simulink model "main"  (R2024a)
settings: Solver=FixedStepDiscrete  StartTime=0.0  StopTime=5  RelTol=1e-3
PreLoadFcn:
  | RTWConfigurationCB('preloadfcn', bdroot);
model workspace (MAT data in the model file):
  fault_count = 0
undefined symbols (not defined in the file or in its folder): Call, Function
libraries: canmsglib x15, c280xlib x13, c2837xDlib x9, c2802xlib x8, simulink x4, slpidlib x1
(part 1 of 2)
settings Model: SimulationMode=external  ExtModeTrigDuration=8  Creator=Brian  LastModifiedBy=benjaminlevin
settings SolverCC: AutoInsertRateTranBlk=on
settings OptimizationCC: DefaultUnderspecifiedDataType=single  EnhancedBackFolding=on  PassReuseOutputArgsAs=Individual arguments  MaxStackSize=1024  OptimizeBlockOrder=speed  DifferentSizesBufferReuse=on  OptimizationCustomize=off  DenormalBehavior=FlushToZero  EfficientTunableParamExpr=on
settings DebuggingCC: ParameterTunabilityLossMsg=error
settings HardwareCC: ProdBitPerChar=16  ProdBitPerInt=16  ProdBitPerPointer=32  ProdBitPerSizeT=32  ProdBitPerPtrDiffT=32  ProdLargestAtomicInteger=Integer  ProdLargestAtomicFloat=None  ProdWordSize=16  ProdLongLongMode=on  ProdHWDeviceType=Texas Instruments->C2000  HardwareBoardFeatureSet=SoCBlockset
settings ModelReferenceCC: EnableRefExpFcnMdlSchedulingChecks=on  ModelReferenceNumInstancesAllowed=Single
settings SFSimCC: MATLABDynamicMemAlloc=off
settings RTWCC: Description=Embedded Coder  SystemTargetFile=ert.tlc  HardwareBoard=TI Delfino F28379D LaunchPad  TemplateMakefile=ert_default_tmf  Toolchain=Texas Instruments Code Composer Studio (C2000)  CodeProfilingSaveOptions=MetricsOnly  GPUComputeCapability=3.5
settings CodeAppCC: ForceParamTrailComments=on  IgnoreCustomStorageClasses=off  OperatorAnnotations=on  SimulinkDataObjDesc=on  SFDataObjDesc=on  InsertBlockDesc=on
settings ERTTargetCC: CodeReplacementLibrary=TI C28x  ExtModeTransport=4  ExtModeStaticAlloc=on  ExtModeAutomaticAllocSize=off  ExtModeStaticAllocSize=10000  ExtModeMexFile=ext_xcp  ExtModeIntrfLevel=Level2 - Open

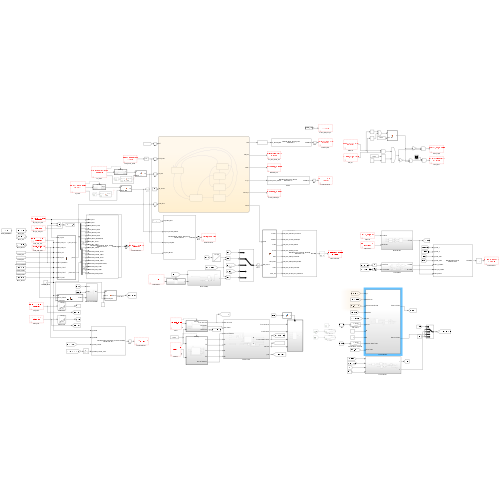
[thumbnail: Simulink's stored preview of the top-level diagram]
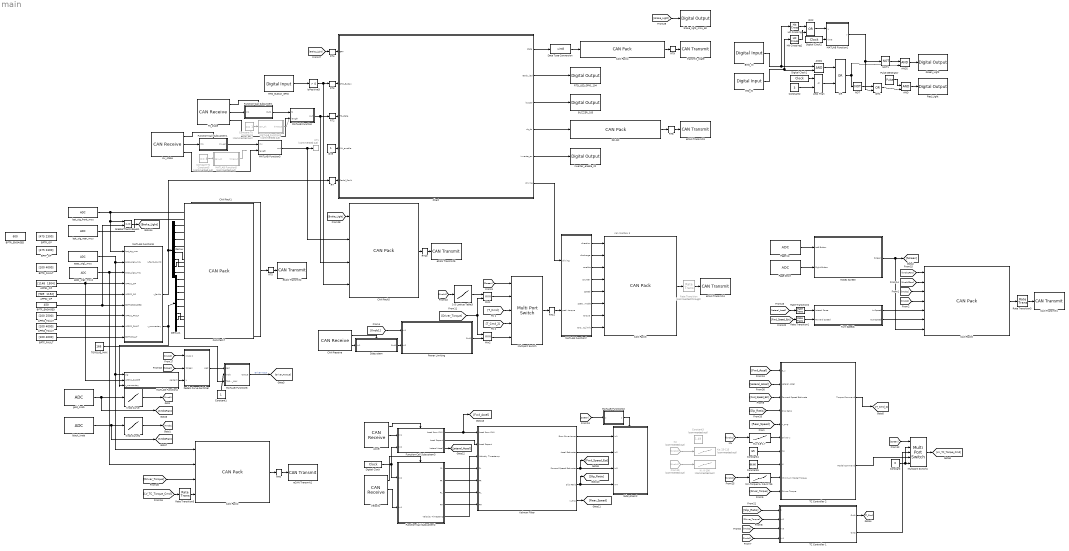
== system main ==
  note: can mailbox 3
  1-D Lookup Table3 : Lookup_n-D  NumberOfTableDimensions=1  BreakpointsForDimension1=[1;10]  Table=[0;166]  ExtrapMethod=Clip  InternalRulePriority=Speed  RndMeth=Simplest
  AND : Logic  IconShape=distinctive  AllPortsSameDT=off  OutDataTypeStr=boolean
  AND1 : Logic  IconShape=distinctive  AllPortsSameDT=off  OutDataTypeStr=boolean
  AND2 : Logic  IconShape=distinctive  AllPortsSameDT=off  OutDataTypeStr=boolean
  APPS1_FAULT : Constant  Value=[100 2500]  VectorParams1D=off
  APPS1_OP : Constant  Value="[1148  1504]"  VectorParams1D=off
  APPS2_FAULT : Constant  Value=[100 4000]  VectorParams1D=off
  APPS2_OP : Constant  Value="[989  1152]"  VectorParams1D=off
  Accel : c280xlib/CAN Receive  chipFamily=C280x  useModule=CAN_B  mailboxNo=10  messageID=52  messageType=Standard (11-bit identifier)  enableAcceptanceFiltering=off  messageIDMask=0  sampleTime=.001  dataType=CAN_MESSAGE_TYPE  outputAction=Output last received values  initValue=0  outputMessageID=off  outputMessageLength=on  outputMessageTimeStamp=off  postInterrupt=off  interruptLine=0
  BMS_IN : c2837xDlib/Digital Input  GPIO_Number=GPIO104~GPIO111  GPIO_Bit0=off  GPIO_Bit1=off  GPIO_Bit2=off  GPIO_Bit3=off  GPIO_Bit4=off  GPIO_Bit5=off  GPIO_Bit6=off  GPIO_Bit7=on  sampleTime=0.1  dataType=auto  GPIO_Bit0_Qualification=Sync to SYSCLKOUT  GPIO_Bit1_Qualification=Sync to SYSCLKOUT  GPIO_Bit2_Qualification=Sync to SYSCLKOUT  GPIO_Bit3_Qualification=Sync to SYSCLKOUT  GPIO_Bit4_Qualification=Sync to SYSCLKOUT  GPIO_Bit5_Qualification=Sync to SYSCLKOUT  GPIO_Bit6_Qualification=Sync to SYSCLKOUT  GPIO_Bit7_Qualification=Sync to SYSCLKOUT  Qualification_Period=-1
  BPTF_ENGAGED : Constant  Value=450  VectorParams1D=off
  BPTF_FAULT : Constant  Value=[100 4000]  VectorParams1D=off
  BPTF_OP : Constant  Value=[475 2300]  VectorParams1D=off
  BPTR_ENGAGED : Constant  Value=600  VectorParams1D=off
  BPTR_FAULT : Constant  Value=[100 4000]  VectorParams1D=off
  BPTR_OP : Constant  Value=[475 2300]  VectorParams1D=off
  BUZZER_105 : c2837xDlib/Digital Output  GPIO_Number=GPIO104~GPIO111  GPIO_Bit0=off  GPIO_BIT0_Toggle=off  GPIO_Bit1=on  GPIO_BIT1_Toggle=off  GPIO_Bit2=off  GPIO_BIT2_Toggle=off  GPIO_Bit3=off  GPIO_BIT3_Toggle=off  GPIO_Bit4=off  GPIO_BIT4_Toggle=off  GPIO_Bit5=off  GPIO_BIT5_Toggle=off  GPIO_Bit6=off  GPIO_BIT6_Toggle=off  GPIO_Bit7=off  GPIO_BIT7_Toggle=off
  CAN Pack1 : canmsglib/CAN Pack  MsgList=(none)  MsgName=M402_Brakes_Faults_Display  MsgIDType=Standard (11-bit identifier)  MsgIdentifier=402  MsgLength=6  Remote=off  ApplyMinMax=off  BusOutput=off  SignalInfo={'LV_BPT_Front','16','16','LE','unsigned','Standard','0','1','0','-Inf','Inf';'LV_BPT_Rear','0','16','LE','unsigned','Standard','0','1','0','-Inf','Inf';'LV_Fault_APPS1_Lower','32','1','LE','unsigned','Standard','0','1','0','0','1';'LV_Fault_APPS1_Upper','33','1','LE','unsigned','Standard','0','1','0','0','1';'LV_Fault_APPS2_Lower','34','1','LE','unsigned','Standard','0','1','0','0','1';'LV_Fault_APPS2_Upper','35','1','LE','unsigned','Standard','0','1','0','0','1';'LV_Fault_APPS_Implausibility','38','1','LE','unsigned','Standard','0','1','0','0','1';'LV_Fault_BPT_Lower','36','1','LE','unsigned','Standard','0','1','0','0','1';'LV_Fault_BPT_Upper','37','1','LE','unsigned','Standard','0','1','0','0','1';'LV_Fault_Both_Pedals','39','1','LE','unsigned','Standard','0','1','0','0','1';'LV_Momentary_APPS1_Lower','40','1','LE','unsigned','Standard','0','1','0','0','1';'LV_Momentary_APPS1_Upper','41','1','LE','unsigned','Standard','0','1','0','0','1';'LV_Momentary_APPS2_Lower','42','1','LE','unsigned','Standard','0','1','0','0','1';'LV_Momentary_APPS2_Upper','43','1','LE','unsigned','Standard','0','1','0','0','1';'LV_Momentary_APPS_Implausibility','46','1','LE','unsigned','Standard','0','1','0','0','1';'LV_Momentary_BPT_Lower','44','1','LE','unsigned','Standard','0','1','0','0','1';'LV_Momentary_BPT_Upper','45','1','LE','unsigned','Standard','0','1','0','0','1';'LV_Momentary_Both_Pedals','47','1','LE','unsigned','Standard','0','1','0','0','1'}
      settings: DataFormat=manually specified signals
  CAN Pack2 : canmsglib/CAN Pack  MsgList=(none)  MsgName=M401_Accelerator_Controls  MsgIDType=Standard (11-bit identifier)  MsgIdentifier=401  MsgLength=8  Remote=off  ApplyMinMax=off  BusOutput=off  SignalInfo={'LV_APPS1','0','16','LE','unsigned','Standard','0','1','0','0','4095';'LV_APPS2','16','16','LE','unsigned','Standard','0','1','0','0','4095';'LV_Driver_Torque','48','16','LE','signed','Standard','0','0.1','0','-3276.8','3276.7';'LV_Kalman_Torque_Cmd','32','16','LE','signed','Standard','0','0.1','0','-3276.8','3276.7'}
      settings: DataFormat=manually specified signals
  CAN Pack3 : canmsglib/CAN Pack  MsgList=(none)  MsgName=M176_Command_Message  MsgIDType=Standard (11-bit identifier)  MsgIdentifier=176  MsgLength=8  Remote=off  ApplyMinMax=off  BusOutput=off  SignalInfo={'VCU_INV_Direction_Command','32','1','LE','unsigned','Standard','0','1','0','0','1';'VCU_INV_Inverter_Discharge','41','1','LE','unsigned','Standard','0','1','0','0','1';'VCU_INV_Inverter_Enable','40','1','LE','unsigned','Standard','0','1','0','0','1';'VCU_INV_Rolling_Counter','44','4','LE','unsigned','Standard','0','1','0','0','15';'VCU_INV_Speed_Command','16','16','LE','signed','Standard','0','1','0','-32768','32767';'VCU_INV_Speed_Mode_Enable','42','1','LE','unsigned','Standard','0','1','0','0','1';'VCU_INV_Torque_Command','0','16','LE','signed','Standard','0','0.1','0','-3276.8','3276.7';'VCU_INV_Torque_Limit_Command','48','16','LE','signed','Standard','0','0.1','0','-3276.8','3276.7'}
      settings: DataFormat=manually specified signals
  CAN Pack4 : canmsglib/CAN Pack  MsgList=(none)  MsgName=M001_Vehicle_State  MsgIDType=Standard (11-bit identifier)  MsgIdentifier=1  MsgLength=1  Remote=off  ApplyMinMax=off  BusOutput=off  SignalInfo={'LV_Vehicle_State','0','8','LE','signed','Standard','0','1','0','-Inf','Inf'}
      settings: DataFormat=manually specified signals
  CAN Pack5 : canmsglib/CAN Pack  MsgList=(none)  MsgName=M403_Vehicle_State_Inputs  MsgIDType=Standard (11-bit identifier)  MsgIdentifier=403  MsgLength=4  Remote=off  ApplyMinMax=off  BusOutput=off  SignalInfo={'LV_Brake_Light','0','8','LE','unsigned','Standard','0','1','0','-Inf','Inf';'LV_Echo_Inverter_Enable','8','8','LE','signed','Standard','0','1','0','-Inf','Inf';'LV_Echo_TS_State','16','8','LE','signed','Standard','0','1','0','-Inf','Inf';'LV_RTD_Button','24','8','LE','unsigned','Standard','0','1','0','-Inf','Inf'}
      settings: DataFormat=manually specified signals
  CAN Pack6 : canmsglib/CAN Pack  MsgList=(none)  MsgName=M053_MoTec  MsgIDType=Standard (11-bit identifier)  MsgIdentifier=53  MsgLength=8  Remote=off  ApplyMinMax=off  BusOutput=off  SignalInfo={'LV_Knob_1','32','8','LE','unsigned','Standard','0','20','0','0','5100';'LV_Knob_2','40','8','LE','unsigned','Standard','0','20','0','0','5100';'LV_Knob_Tick1','12','4','LE','unsigned','Standard','0','1','0','0','15';'LV_Knob_Tick2','28','4','LE','unsigned','Standard','0','1','0','0','15';'MoTec_In_Speed','0','12','LE','unsigned','Standard','0','0.1','0','0','409.5';'MoTec_Out_Speed','16','12','LE','unsigned','Standard','0','0.1','0','0','409.5';'MoTec_Screen','48','8','LE','unsigned','Standard','0','1','0','0','255'}
      settings: LibrarySourceBlock=c2000lib/Target Communication/CAN Pack  DataFormat=manually specified signals
  CAN Pack7 : canmsglib/CAN Pack  MsgList=(none)  MsgName=M402_Brakes_Faults_Display  MsgIDType=Standard (11-bit identifier)  MsgIdentifier=402  MsgLength=6  Remote=off  ApplyMinMax=off  BusOutput=off  SignalInfo={'LV_BPT_Front','16','16','LE','unsigned','Standard','0','1','0','-Inf','Inf';'LV_BPT_Rear','0','16','LE','unsigned','Standard','0','1','0','-Inf','Inf';'LV_Fault_APPS1_Lower','32','1','LE','unsigned','Standard','0','1','0','0','1';'LV_Fault_APPS1_Upper','33','1','LE','unsigned','Standard','0','1','0','0','1';'LV_Fault_APPS2_Lower','34','1','LE','unsigned','Standard','0','1','0','0','1';'LV_Fault_APPS2_Upper','35','1','LE','unsigned','Standard','0','1','0','0','1';'LV_Fault_APPS_Implausibility','38','1','LE','unsigned','Standard','0','1','0','0','1';'LV_Fault_BPT_Lower','36','1','LE','unsigned','Standard','0','1','0','0','1';'LV_Fault_BPT_Upper','37','1','LE','unsigned','Standard','0','1','0','0','1';'LV_Fault_Both_Pedals','39','1','LE','unsigned','Standard','0','1','0','0','1';'LV_Momentary_APPS1_Lower','40','1','LE','unsigned','Standard','0','1','0','0','1';'LV_Momentary_APPS1_Upper','41','1','LE','unsigned','Standard','0','1','0','0','1';'LV_Momentary_APPS2_Lower','42','1','LE','unsigned','Standard','0','1','0','0','1';'LV_Momentary_APPS2_Upper','43','1','LE','unsigned','Standard','0','1','0','0','1';'LV_Momentary_APPS_Implausibility','46','1','LE','unsigned','Standard','0','1','0','0','1';'LV_Momentary_BPT_Lower','44','1','LE','unsigned','Standard','0','1','0','0','1';'LV_Momentary_BPT_Upper','45','1','LE','unsigned','Standard','0','1','0','0','1';'LV_Momentary_Both_Pedals','47','1','LE','unsigned','Standard','0','1','0','0','1'}
      settings: DataFormat=manually specified signals
  CAN Receive : c280xlib/CAN Receive  chipFamily=C280x  useModule=CAN_B  mailboxNo=14  messageID=149  messageType=Standard (11-bit identifier)  enableAcceptanceFiltering=off  messageIDMask=0  sampleTime=0.01  dataType=CAN_MESSAGE_TYPE  outputAction=Output last received values  initValue=0  outputMessageID=off  outputMessageLength=off  outputMessageTimeStamp=off  postInterrupt=off  interruptLine=0
  CAN Transmit1 : c280xlib/CAN Transmit  chipFamily=C280x  useModule=CAN_B  mailboxNo=12  messageID=53  messageType=Standard (11-bit identifier)  enableBlockingMode=off  postInterrupt=off  interruptLine=0
  Chart : Stateflow chart  TreatAsAtomicUnit=on  SystemSampleTime=0.01
      settings: RTWSystemCode=Inline  RTWFcnNameOpts=Use subsystem name  RTWFileNameOpts=Use subsystem name  PortSchema="{\"entries\":[{\"content\":{\"sides\":[{\"content\":{\"connectorIds\":[\"In1\",\"In2\",\"In5\",\"In4\",\"In3\"]},\"type\":\"ConnectorPlacement.EquallySpacedRectSide\",\"uuid\":\"e489c846-491e-4e82-9c5f-b669d7c96954\"},{\"content\":{\"connectorIds\":[\"Out1\",\"Out2\",\"Out3\",\"Out4\",\"Out5\",\"Out6\"],\"side\":\"RIGHT\"},\"type\":\"ConnectorPlacement.EquallySpacedRectSide\",\"uuid\":\"cbb46da5-6eb6-44f9-baf3-a24ec6c96225\"},{\"content\":{\"side\":\"TOP\"},\"type\":\"ConnectorPlacement.EquallySpacedRectSide\",\"uuid\":\"c6202e3b-aafb-4b81-a309-4cc98c9bb853\"},{\"content\":{\"side\":\"BOTTOM\"},\"type\":\"ConnectorPlacement.EquallySpacedRectSide\",\"uuid\":\"d6a20d7c-ea9b-4afd-8884-952a45f498ea\"}]},\"type\":\"ConnectorPlacement.EquallySpacedConnector\",\"uuid\":\"7c3bea70-19b9-40c4-b7cb-79b1c3f0d3c0\"}],\"packageUris\":[\"http://schema.mathworks.com/mf0/Connector/R2020b\"],\"version\":\"1.0\"}"
  Compare To Constant4 : simulink/Logic and Bit Operations/Compare To Constant  Commented=on  relop===  const=1  OutDataTypeStr=boolean
  Compare To Constant5 : simulink/Logic and Bit Operations/Compare To Constant  Commented=on  relop===  const=8  OutDataTypeStr=boolean
  Constant : Constant  Value=0
  Constant1 : Constant
  Constant2 : Constant  Value=3
  Constant3 : Constant  Commented=on  Value=1.49
  Constant4 : Constant  Value=65
  Constant5 : Constant  Value=66.66
  DC-DC : canmsglib/CAN Pack  MsgList=(none)  MsgName=M003_DCDC_Enable  MsgIDType=Standard (11-bit identifier)  MsgIdentifier=3  MsgLength=1  Remote=off  ApplyMinMax=off  BusOutput=off  SignalInfo={'LV_ACC_DCDC_Enable','0','8','LE','signed','Standard','0','1','0','-Inf','Inf'}
      settings: DataFormat=manually specified signals
  Data Type Conversion : DataTypeConversion  OutDataTypeStr=uint8  SaturateOnIntegerOverflow=off  RndMeth=Floor
  Demux : Demux  Outputs=8
  Demux1 : Demux  Outputs=8
  Digital Clock : DigitalClock  SampleTime=0.001
  Digital Clock1 : DigitalClock  SampleTime=0.1
  Digital Clock2 : DigitalClock  SampleTime=0.1
  From19 : From  Commented=on  GotoTag=Knob1
  Function-Call Subsystem : Subsystem  TreatAsAtomicUnit=on
  Function-Call Subsystem1 : Subsystem  TreatAsAtomicUnit=on
  Function-Call Subsystem2 : Subsystem  TreatAsAtomicUnit=on
  Function-Call Subsystem3 : Subsystem  TreatAsAtomicUnit=on
  GreaterThanOrEqual1 : RelationalOperator  OutDataTypeStr=boolean  RndMeth=Simplest  InputSameDT=off
  Green_Light : c2837xDlib/Digital Output  GPIO_Number=GPIO16~GPIO23  GPIO_Bit0=off  GPIO_BIT0_Toggle=off  GPIO_Bit1=off  GPIO_BIT1_Toggle=off  GPIO_Bit2=on  GPIO_BIT2_Toggle=off  GPIO_Bit3=off  GPIO_BIT3_Toggle=off  GPIO_Bit4=off  GPIO_BIT4_Toggle=off  GPIO_Bit5=off  GPIO_BIT5_Toggle=off  GPIO_Bit6=off  GPIO_BIT6_Toggle=off  GPIO_Bit7=off  GPIO_BIT7_Toggle=off
  Hit Crossing : HitCross  HitCrossingOffset=0.5  HitCrossingDirection=rising
  Hit Crossing1 : HitCross  HitCrossingOffset=0.5  HitCrossingDirection=rising
  IMD_IN : c2837xDlib/Digital Input  GPIO_Number=GPIO64~GPIO71  GPIO_Bit0=off  GPIO_Bit1=off  GPIO_Bit2=off  GPIO_Bit3=on  GPIO_Bit4=off  GPIO_Bit5=off  GPIO_Bit6=off  GPIO_Bit7=off  sampleTime=0.1  dataType=auto  GPIO_Bit0_Qualification=Sync to SYSCLKOUT  GPIO_Bit1_Qualification=Sync to SYSCLKOUT  GPIO_Bit2_Qualification=Sync to SYSCLKOUT  GPIO_Bit3_Qualification=Sync to SYSCLKOUT  GPIO_Bit4_Qualification=Sync to SYSCLKOUT  GPIO_Bit5_Qualification=Sync to SYSCLKOUT  GPIO_Bit6_Qualification=Sync to SYSCLKOUT  GPIO_Bit7_Qualification=Sync to SYSCLKOUT  Qualification_Period=-1
  IsPositive3 : simulink/Logic and Bit Operations/Compare To Zero  relop=>  OutDataTypeStr=boolean
  Kalman Filter : Subsystem
  "Ki: 0-100 " : Lookup_n-D  Commented=on  NumberOfTableDimensions=1  BreakpointsForDimension1=[1 10]  Table=[0 100]  ExtrapMethod=Clip  InternalRulePriority=Speed  RndMeth=Simplest
  Knob Curve : Lookup_n-D  NumberOfTableDimensions=1  BreakpointsForDimension1=[0;178;680;1180;1675;2199;2692;3170;3690;4095]  BreakpointsForDimension1DataTypeStr=uint16  BeginIndexSearchUsingPreviousIndexResult=on  Table=[1;2;3;4;5;6;7;8;9;10]  TableDataTypeStr=double  InterpMethod=Nearest  ExtrapMethod=Clip  DiagnosticForOutOfRangeInput=Warning  UseLastTableValue=on  InternalRulePriority=Speed  OutDataTypeStr=double  RndMeth=Simplest
  Knob Curve1 : Lookup_n-D  NumberOfTableDimensions=1  BreakpointsForDimension1=[0;110;616;1132;1645;2160;2668;3175;3680;4095]  BreakpointsForDimension1DataTypeStr=uint16  BeginIndexSearchUsingPreviousIndexResult=on  Table=[1;2;3;4;5;6;7;8;9;10]  TableDataTypeStr=double  InterpMethod=Nearest  ExtrapMethod=Clip  DiagnosticForOutOfRangeInput=Warning  UseLastTableValue=on  InternalRulePriority=Speed  OutDataTypeStr=double  RndMeth=Simplest
  Kp : From  Commented=on  GotoTag=Knob2
  Kp: 25-115 : Lookup_n-D  Commented=on  NumberOfTableDimensions=1  BreakpointsForDimension1=[1 10]  Table=[25 115]  InternalRulePriority=Speed  RndMeth=Simplest
  Less Than : RelationalOperator  Operator=<  OutDataTypeStr=boolean  RndMeth=Simplest  InputSameDT=off
  MATLAB Function : MATLAB Function  TreatAsAtomicUnit=on
  MATLAB Function1 : MATLAB Function  TreatAsAtomicUnit=on
  MATLAB Function10 : MATLAB Function  TreatAsAtomicUnit=on
  MATLAB Function2 : MATLAB Function  Commented=on  TreatAsAtomicUnit=on
  MATLAB Function3 : MATLAB Function  TreatAsAtomicUnit=on
  MATLAB Function4 : MATLAB Function  TreatAsAtomicUnit=on
  MATLAB Function5 : MATLAB Function  Commented=on  TreatAsAtomicUnit=on
  MATLAB Function6 : MATLAB Function  TreatAsAtomicUnit=on
  MATLAB Function7 : MATLAB Function  TreatAsAtomicUnit=on
  MATLAB Function9 : MATLAB Function  TreatAsAtomicUnit=on
  Min Torque %: 0.5-0.725 : Lookup_n-D  NumberOfTableDimensions=1  BreakpointsForDimension1=[1 10]  Table=[0.5 0.725]  InternalRulePriority=Speed  RndMeth=Simplest
  Min1 : MinMax  Inputs=2
  Min2 : MinMax  Inputs=2
  Motec Screen : Subsystem
  Mu: 0.8-1.7 : Lookup_n-D  NumberOfTableDimensions=1  BreakpointsForDimension1=[1 10]  Table=[0.8 1.7]  ExtrapMethod=Clip  InternalRulePriority=Speed  RndMeth=Simplest
  Multiport Switch : MultiPortSwitch  DataPortOrder=Zero-based contiguous  DataPortForDefault=Additional data port  zeroidx=on  SaturateOnIntegerOverflow=off  InputSameDT=off
  Multiport Switch1 : MultiPortSwitch  DataPortOrder=Zero-based contiguous  DataPortForDefault=Additional data port  zeroidx=on  SaturateOnIntegerOverflow=off  InputSameDT=off
  NOT : Logic  Operator=NOT  IconShape=distinctive  AllPortsSameDT=off  OutDataTypeStr=boolean
  NOT1 : Logic  Operator=NOT  IconShape=distinctive  AllPortsSameDT=off  OutDataTypeStr=boolean
  OR : Logic  Operator=OR  IconShape=distinctive  AllPortsSameDT=off  OutDataTypeStr=boolean
  OR1 : Logic  Operator=OR  IconShape=distinctive  AllPortsSameDT=off  OutDataTypeStr=boolean
  OR2 : Logic  Operator=OR  IconShape=distinctive  AllPortsSameDT=off  OutDataTypeStr=boolean
  One : Constant  OutDataTypeStr=Inherit: Inherit via back propagation
  Page Down : c2802xlib/ADC  blkParamProc=C2000_Type4  ADCModule=A  samplingMode=Single sample mode  ADCResolution=12-bit (Single-ended input)  useSOC1=SOC6  useSOC2=SOC0_SOC1  SOCAcquisitionWindow=60  SOCTriggerSource=Software  SOCInterruptTrigger=No ADCINT  Ts=0.01  dType=uint16  postInterrupt=off  interruptSel=ADCINT1  ADCINTContinuous=on  endma=off  chdma=1  conv1=ADCINA0  conv2=ADCINA0 and ADCINB0  conv1_Type4=ADCIN0  conv2_Type4=ADCIN0 and ADCIN1
  Page Up : c2802xlib/ADC  blkParamProc=C2000_Type4  ADCModule=A  samplingMode=Single sample mode  ADCResolution=12-bit (Single-ended input)  useSOC1=SOC7  useSOC2=SOC0_SOC1  SOCAcquisitionWindow=60  SOCTriggerSource=Software  SOCInterruptTrigger=No ADCINT  Ts=0.01  dType=uint16  postInterrupt=off  interruptSel=ADCINT1  ADCINTContinuous=on  endma=off  chdma=1  conv1=ADCINA0  conv2=ADCINA0 and ADCINB0  conv1_Type4=ADCIN2  conv2_Type4=ADCIN0 and ADCIN1
  Pedals Curve Switcher : Subsystem
  Power Limiting : Subsystem
  Pulse Generator : DiscretePulseGenerator  PulseType=Time based  Period=0.33  PulseWidth=50
  RT{,2..4,6} (5 alike) : RateTransition  OutPortSampleTime=0.01
  RT1 : RateTransition  Commented=on  OutPortSampleTime=0.01
  RT10 : RateTransition  OutPortSampleTime=.1
  RT11 : RateTransition  OutPortSampleTime=.01
  RT5 : RateTransition  OutPortSampleTime=.1
  RT8 : RateTransition  OutPortSampleTime=.5
  RT9 : RateTransition  OutPortSampleTime=.5
  RTD_Button_GPIO : c2837xDlib/Digital Input  GPIO_Number=GPIO32~GPIO39  GPIO_Bit0=on  GPIO_Bit1=off  GPIO_Bit2=off  GPIO_Bit3=off  GPIO_Bit4=off  GPIO_Bit5=off  GPIO_Bit6=off  GPIO_Bit7=off  sampleTime=0.1  dataType=uint8  GPIO_Bit0_Qualification=Sync to SYSCLKOUT  GPIO_Bit1_Qualification=Sync to SYSCLKOUT  GPIO_Bit2_Qualification=Sync to SYSCLKOUT  GPIO_Bit3_Qualification=Sync to SYSCLKOUT  GPIO_Bit4_Qualification=Sync to SYSCLKOUT  GPIO_Bit5_Qualification=Sync to SYSCLKOUT  GPIO_Bit6_Qualification=Sync to SYSCLKOUT  GPIO_Bit7_Qualification=Sync to SYSCLKOUT  Qualification_Period=-1
  RTD_LED_GPIO_104 : c2837xDlib/Digital Output  GPIO_Number=GPIO104~GPIO111  GPIO_Bit0=on  GPIO_BIT0_Toggle=off  GPIO_Bit1=off  GPIO_BIT1_Toggle=off  GPIO_Bit2=off  GPIO_BIT2_Toggle=off  GPIO_Bit3=off  GPIO_BIT3_Toggle=off  GPIO_Bit4=off  GPIO_BIT4_Toggle=off  GPIO_Bit5=off  GPIO_BIT5_Toggle=off  GPIO_Bit6=off  GPIO_BIT6_Toggle=off  GPIO_Bit7=off  GPIO_BIT7_Toggle=off
  Rate Transition : RateTransition  Commented=through  OutPortSampleTime=0.003
  Rate Transition1 : RateTransition  OutPortSampleTime=0.01
  Rate Transition2 : RateTransition  OutPortSampleTime=0.01
  Rate Transition3 : RateTransition  OutPortSampleTime=0.5
  Rate Transition5 : RateTransition  OutPortSampleTime=0.01
  Red_Light : c2837xDlib/Digital Output  GPIO_Number=GPIO16~GPIO23  GPIO_Bit0=off  GPIO_BIT0_Toggle=off  GPIO_Bit1=off  GPIO_BIT1_Toggle=off  GPIO_Bit2=off  GPIO_BIT2_Toggle=off  GPIO_Bit3=on  GPIO_BIT3_Toggle=off  GPIO_Bit4=off  GPIO_BIT4_Toggle=off  GPIO_Bit5=off  GPIO_BIT5_Toggle=off  GPIO_Bit6=off  GPIO_BIT6_Toggle=off  GPIO_Bit7=off  GPIO_BIT7_Toggle=off
  Subsystem : Subsystem
  Subsystem2 : Subsystem
  TC Controller 1 : Subsystem
  TC Controller 2 : Subsystem
  TORQUE_MAX : Constant  Value=166
  TS_state : c280xlib/CAN Receive  chipFamily=C280x  useModule=CAN_B  mailboxNo=2  messageID=2  messageType=Standard (11-bit identifier)  enableAcceptanceFiltering=off  messageIDMask=0  sampleTime=.25  dataType=CAN_MESSAGE_TYPE  outputAction=Reset all fields to zero  initValue=0  outputMessageID=off  outputMessageLength=on  outputMessageTimeStamp=off  postInterrupt=off  interruptLine=0
  Turn Speeds : Subsystem
  Velocity : c280xlib/CAN Receive  chipFamily=C280x  useModule=CAN_B  mailboxNo=9  messageID=51  messageType=Standard (11-bit identifier)  enableAcceptanceFiltering=off  messageIDMask=0  sampleTime=.001  dataType=CAN_MESSAGE_TYPE  outputAction=Output last received values  initValue=0  outputMessageID=off  outputMessageLength=on  outputMessageTimeStamp=off  postInterrupt=off  interruptLine=0
  apps_sig1_mcu : c2802xlib/ADC  blkParamProc=C2000_Type4  ADCModule=A  samplingMode=Single sample mode  ADCResolution=12-bit (Single-ended input)  useSOC1=SOC15  useSOC2=SOC0_SOC1  SOCAcquisitionWindow=60  SOCTriggerSource=Software  SOCInterruptTrigger=No ADCINT  Ts=0.01  dType=uint16  postInterrupt=off  interruptSel=ADCINT1  ADCINTContinuous=on  endma=off  chdma=1  conv1=ADCINA0  conv2=ADCINA0 and ADCINB0  conv1_Type4=ADCIN3  conv2_Type4=ADCIN0 and ADCIN1
  apps_sig2_mcu1 : c2802xlib/ADC  blkParamProc=C2000_Type4  ADCModule=C  samplingMode=Single sample mode  ADCResolution=12-bit (Single-ended input)  useSOC1=SOC10  useSOC2=SOC0_SOC1  SOCAcquisitionWindow=60  SOCTriggerSource=Software  SOCInterruptTrigger=No ADCINT  Ts=0.01  dType=uint16  postInterrupt=off  interruptSel=ADCINT1  ADCINTContinuous=on  endma=off  chdma=1  conv1=ADCINA0  conv2=ADCINA0 and ADCINB0  conv1_Type4=ADCIN2  conv2_Type4=ADCIN0 and ADCIN1
  black_knob : c2802xlib/ADC  blkParamProc=C2000_Type4  ADCModule=A  samplingMode=Single sample mode  ADCResolution=12-bit (Single-ended input)  useSOC1=SOC10  useSOC2=SOC0_SOC1  SOCAcquisitionWindow=60  SOCTriggerSource=Software  SOCInterruptTrigger=No ADCINT  Ts=0.01  dType=uint16  postInterrupt=off  interruptSel=ADCINT1  ADCINTContinuous=on  endma=off  chdma=1  conv1=ADCINA0  conv2=ADCINA0 and ADCINB0  conv1_Type4=ADCIN14  conv2_Type4=ADCIN0 and ADCIN1
  bpt_sig_front_mcu : c2802xlib/ADC  blkParamProc=C2000_Type4  ADCModule=B  samplingMode=Single sample mode  ADCResolution=12-bit (Single-ended input)  useSOC1=SOC6  useSOC2=SOC0_SOC1  SOCAcquisitionWindow=60  SOCTriggerSource=Software  SOCInterruptTrigger=No ADCINT  Ts=0.01  dType=uint16  postInterrupt=off  interruptSel=ADCINT1  ADCINTContinuous=on  endma=off  chdma=1  conv1=ADCINA0  conv2=ADCINA0 and ADCINB0  conv1_Type4=ADCIN3  conv2_Type4=ADCIN0 and ADCIN1
  bpt_sig_rear_mcu : c2802xlib/ADC  blkParamProc=C2000_Type4  ADCModule=C  samplingMode=Single sample mode  ADCResolution=12-bit (Single-ended input)  useSOC1=SOC6  useSOC2=SOC0_SOC1  SOCAcquisitionWindow=60  SOCTriggerSource=Software  SOCInterruptTrigger=No ADCINT  Ts=0.01  dType=uint16  postInterrupt=off  interruptSel=ADCINT1  ADCINTContinuous=on  endma=off  chdma=1  conv1=ADCINA0  conv2=ADCINA0 and ADCINB0  conv1_Type4=ADCIN3  conv2_Type4=ADCIN0 and ADCIN1
  brake_light_mcu_60 : c2837xDlib/Digital Output  GPIO_Number=GPIO56~GPIO63  GPIO_Bit0=off  GPIO_BIT0_Toggle=off  GPIO_Bit1=off  GPIO_BIT1_Toggle=off  GPIO_Bit2=off  GPIO_BIT2_Toggle=off  GPIO_Bit3=off  GPIO_BIT3_Toggle=off  GPIO_Bit4=on  GPIO_BIT4_Toggle=off  GPIO_Bit5=off  GPIO_BIT5_Toggle=off  GPIO_Bit6=off  GPIO_BIT6_Toggle=off  GPIO_Bit7=off  GPIO_BIT7_Toggle=off
  eCAN Transmit1 : c280xlib/CAN Transmit  chipFamily=C280x  useModule=CAN_B  mailboxNo=6  messageID=401  messageType=Standard (11-bit identifier)  enableBlockingMode=off  postInterrupt=off  interruptLine=0
  eCAN Transmit2 : c280xlib/CAN Transmit  chipFamily=C280x  useModule=CAN_B  mailboxNo=7  messageID=402  messageType=Standard (11-bit identifier)  enableBlockingMode=off  postInterrupt=off  interruptLine=0
  eCAN Transmit3 : c280xlib/CAN Transmit  chipFamily=C280x  useModule=CAN_B  mailboxNo=3  messageID=3  messageType=Standard (11-bit identifier)  enableBlockingMode=off  postInterrupt=off  interruptLine=0
  eCAN Transmit4 : c280xlib/CAN Transmit  chipFamily=C280x  useModule=CAN_B  mailboxNo=4  messageID=192  messageType=Standard (11-bit identifier)  enableBlockingMode=off  postInterrupt=off  interruptLine=0
  eCAN Transmit5 : c280xlib/CAN Transmit  chipFamily=C280x  useModule=CAN_B  mailboxNo=8  messageID=403  messageType=Standard (11-bit identifier)  enableBlockingMode=off  postInterrupt=off  interruptLine=0
  gold_knob : c2802xlib/ADC  blkParamProc=C2000_Type4  ADCModule=B  samplingMode=Single sample mode  ADCResolution=12-bit (Single-ended input)  useSOC1=SOC10  useSOC2=SOC0_SOC1  SOCAcquisitionWindow=60  SOCTriggerSource=Software  SOCInterruptTrigger=No ADCINT  Ts=0.01  dType=uint16  postInterrupt=off  interruptSel=ADCINT1  ADCINTContinuous=on  endma=off  chdma=1  conv1=ADCINA0  conv2=ADCINA0 and ADCINB0  conv1_Type4=ADCIN2  conv2_Type4=ADCIN0 and ADCIN1
  inv_state : c280xlib/CAN Receive  chipFamily=C280x  useModule=CAN_B  mailboxNo=5  messageID=154  messageType=Standard (11-bit identifier)  enableAcceptanceFiltering=off  messageIDMask=0  sampleTime=.25  dataType=CAN_MESSAGE_TYPE  outputAction=Reset all fields to zero  initValue=0  outputMessageID=off  outputMessageLength=on  outputMessageTimeStamp=off  postInterrupt=off  interruptLine=0
  inverter_enable_22 : c2837xDlib/Digital Output  GPIO_Number=GPIO16~GPIO23  GPIO_Bit0=off  GPIO_BIT0_Toggle=off  GPIO_Bit1=off  GPIO_BIT1_Toggle=off  GPIO_Bit2=off  GPIO_BIT2_Toggle=off  GPIO_Bit3=off  GPIO_BIT3_Toggle=off  GPIO_Bit4=off  GPIO_BIT4_Toggle=off  GPIO_Bit5=off  GPIO_BIT5_Toggle=off  GPIO_Bit6=on  GPIO_BIT6_Toggle=off  GPIO_Bit7=off  GPIO_BIT7_Toggle=off
  transmit_state : c280xlib/CAN Transmit  chipFamily=C280x  useModule=CAN_B  mailboxNo=1  messageID=1  messageType=Standard (11-bit identifier)  enableBlockingMode=off  postInterrupt=off  interruptLine=0
  wires:
  Data Type Conversion/1 -> CAN Pack4/1
  TS_state/2 -> Function-Call Subsystem/1(In1)
  Function-Call Subsystem/1(Out1) -> MATLAB Function/1(ts)
  TS_state/1 -> Function-Call Subsystem/Trigger
  CAN Pack4/1 -> RT9/1
  bpt_sig_rear_mcu/1 -> CAN Pack1/2
  apps_sig1_mcu/1 -> CAN Pack2/1, MATLAB Function4/1(sig), MATLAB Function9/2(apps_sig1_mcu)
  apps_sig2_mcu1/1 -> CAN Pack2/2, MATLAB Function9/3(apps_sig2_mcu)
  RTD_Button_GPIO/1 -> IsPositive3/1
  CAN Pack1/1 -> RT5/1
  gold_knob/1 -> [Knob1Raw], Knob Curve/1
  DC-DC/1 -> RT8/1
  Chart/1(state) -> Data Type Conversion/1
  bpt_sig_front_mcu/1 -> GreaterThanOrEqual1/1, MATLAB Function9/1(bpt_sig_mcu), CAN Pack1/1
  TS_state/3 -> MATLAB Function/2(length)
  Compare To Constant4/1 -> MATLAB Function2/1(can_ok)
  MATLAB Function2/1(timeout) -> ?
  inv_state/1 -> Function-Call Subsystem1/Trigger
  inv_state/2 -> Function-Call Subsystem1/1(In1)
  inv_state/3 -> MATLAB Function3/2(length)
  Compare To Constant5/1 -> MATLAB Function5/1(can_ok)
  Function-Call Subsystem1/1(inv_en) -> MATLAB Function3/1(inv)
  MATLAB Function5/1(timeout) -> ?
  Chart/3(buzzer) -> BUZZER_105/1
  Chart/4(dc_dc) -> DC-DC/1
  Chart/5(inverter_en) -> inverter_enable_22/1
  Chart/6(driving) -> MATLAB Function7/1(driving)
  MATLAB Function7/1(direction) -> CAN Pack3/1
  MATLAB Function7/2(discharge) -> CAN Pack3/2
  MATLAB Function7/3(enable) -> CAN Pack3/3
  MATLAB Function7/5(speed) -> CAN Pack3/5
  MATLAB Function7/4(counter) -> CAN Pack3/4
  MATLAB Function7/6(speed_mode) -> CAN Pack3/6
  MATLAB Function7/7(torque) -> CAN Pack3/7
  MATLAB Function7/8(torque_limit) -> CAN Pack3/8
  Chart/2(ready_led) -> RTD_LED_GPIO_104/1
  IsPositive3/1 -> CAN Pack5/4, RT3/1
  MATLAB Function/1(out) -> CAN Pack5/3, RT2/1
  RT/1 -> Chart/3(Pedal_Fault)
  RT2/1 -> Chart/5(TS_state)
  RT3/1 -> Chart/2(RTD_Button)
  RT4/1 -> Chart/1(BPT)
  MATLAB Function3/1(out) -> RT1/1, CAN Pack5/2
  RT5/1 -> eCAN Transmit2/1
  CAN Pack3/1 -> Rate Transition/1
  RT8/1 -> eCAN Transmit3/1
  RT9/1 -> transmit_state/1
  CAN Pack5/1 -> RT10/1
  RT10/1 -> eCAN Transmit5/1
  RT11/1 -> MATLAB Function7/2(pedal_torque)
  One/1 -> Chart/4(INV_enable)
  APPS1_OP/1 -> MATLAB Function9/4(APPS1_OP), MATLAB Function4/2(APPS1_RANGE)
  APPS2_OP/1 -> MATLAB Function9/5(APPS2_OP)
  APPS1_FAULT/1 -> MATLAB Function9/7(APPS1_FAULT)
  APPS2_FAULT/1 -> MATLAB Function9/8(APPS2_FAULT)
  TORQUE_MAX/1 -> MATLAB Function6/3(TORQUE_MAX)
  BPTF_ENGAGED/1 -> MATLAB Function9/6(BPTF_ENGAGED), GreaterThanOrEqual1/2
  BPTF_FAULT/1 -> MATLAB Function9/9(BPTF_FAULT)
  Demux/1 -> CAN Pack1/3
  Demux/2 -> CAN Pack1/4
  Demux/3 -> CAN Pack1/5
  Demux/4 -> CAN Pack1/6
  Demux/5 -> CAN Pack1/8
  Demux/6 -> CAN Pack1/9
  Demux/7 -> CAN Pack1/7
  Demux/8 -> CAN Pack1/10
  Demux1/1 -> CAN Pack1/11
  Demux1/2 -> CAN Pack1/12
  MATLAB Function9/3(r_momentary) -> MATLAB Function4/3(r_momentary), Demux1/1
  Demux1/3 -> CAN Pack1/13
  Demux1/4 -> CAN Pack1/14
  Demux1/5 -> CAN Pack1/16
  Demux1/6 -> CAN Pack1/17
  Demux1/7 -> CAN Pack1/15
  Demux1/8 -> CAN Pack1/18
  BMS_IN/1 -> Hit Crossing/1, AND1/1
  IMD_IN/1 -> Hit Crossing1/1, AND1/2
  Function-Call Subsystem2/5(Velocity Timestamp) -> Kalman Filter/3(Velocity Timestamp)
  Velocity/1 -> Function-Call Subsystem2/Trigger
  Accel/1 -> Function-Call Subsystem3/Trigger
  Function-Call Subsystem3/2(Accel Report) -> Kalman Filter/2(Accel Report)
  Velocity/2 -> Function-Call Subsystem2/2(In1)
  Function-Call Subsystem2/1(FL) -> Kalman Filter/4(FL)
  Function-Call Subsystem2/3(RL) -> Kalman Filter/6(RL)
  MATLAB Function6/1(torque) -> [Driver_Torque]  "Driver Input"
  Function-Call Subsystem2/4(RR) -> Kalman Filter/7(RR)
  Accel/2 -> Function-Call Subsystem3/1(In1)
  Rate Transition/1 -> eCAN Transmit4/1
  Motec Screen/1(Screen) -> [Screen], CAN Pack6/7
  Function-Call Subsystem3/3(Lateral Accel) -> [Lateral_Accel]
  Turn Speeds/1(In-Speed) -> CAN Pack6/5
  Turn Speeds/2(Out-Speed) -> CAN Pack6/6
  CAN Pack6/1 -> Rate Transition3/1
  Page Down/1 -> Motec Screen/2(Right Button)
  Rate Transition1/1 -> Turn Speeds/2(Forward Speed)
  Rate Transition2/1 -> Turn Speeds/1(Lateral Force)
  Function-Call Subsystem2/2(FR) -> Kalman Filter/5(FR)
  Digital Clock/1 -> Function-Call Subsystem2/1(In2), Function-Call Subsystem3/2(In2)
  Kalman Filter/5(v_avg) -> [Rear_Speed]
  black_knob/1 -> Knob Curve1/1, [Knob2Raw]
  Knob Curve/1 -> [Knob1]
  Constant1/1 -> MATLAB Function6/2(knob)
  Kp/1 -> Kp: 25-115/1
  [Knob1] -> CAN Pack6/3
  Knob Curve1/1 -> [Knob2]
  [Knob2] -> CAN Pack6/4
  [Screen] -> Multiport Switch/1
  [Knob1] -> Mu: 0.8-1.7/1
  [Driver_Torque] -> TC Controller 1/2(In2)
  [Knob1] -> 1-D Lookup Table3/1
  1-D Lookup Table3/1 -> Min1/1
  Min1/1 -> Multiport Switch/2
  [T_Cmd] -> Multiport Switch/3
  [T_Cmd_2] -> Multiport Switch/4
  Multiport Switch/1 -> RT11/1
  Function-Call Subsystem3/1(Accel from CAN) -> [Fwd_Accel], Kalman Filter/1(Accel from CAN)
  Page Up/1 -> Motec Screen/1(Left Button)
  CAN Pack2/1 -> RT6/1
  RT6/1 -> eCAN Transmit1/1
  CAN Receive/2 -> Subsystem/1(In1)
  CAN Receive/1 -> Subsystem/Trigger
  Min2/1 -> Multiport Switch/5
  [Driver_Torque] -> Min2/1, Min1/2
  [Screen] -> Multiport Switch1/1
  Constant/1 -> Multiport Switch1/2, Multiport Switch1/5
  Rate Transition3/1 -> CAN Transmit1/1
  Digital Clock1/1 -> Less Than/1
  Constant2/1 -> Less Than/2
  AND1/1 -> OR/1
  Less Than/1 -> OR/2
  OR/1 -> AND2/2, NOT/1
  Kalman Filter/3(Forward Speed Estimate) -> [Fwd_Speed_Est], Subsystem2/3(In3)
  [Knob2] -> TC Controller 1/3(In3)
  TC Controller 1/1(Out1) -> [T_Cmd]
  TC Controller 1/2(Out2) -> Multiport Switch1/3
  [Knob1] -> TC Controller 1/4(In1)
  Kalman Filter/1(Error Covariance) -> Subsystem2/1(In1)
  Kalman Filter/2(Accel Estimate) -> Subsystem2/2(In2)
  [Screen] -> MATLAB Function10/1(u)
  TC Controller 2/2(Model Command) -> Multiport Switch1/4
  TC Controller 2/1(Torque Command) -> [T_Cmd_2]
  MATLAB Function10/1(y) -> Subsystem2/Enable
  MATLAB Function4/1(percent) -> Pedals Curve Switcher/3(u)
  Pedals Curve Switcher/1(ped) -> MATLAB Function6/1(ped)
  [Driver_Torque] -> TC Controller 2/10(Driver Torque)
  [Knob2Raw] -> CAN Pack6/2
  [Knob1Raw] -> CAN Pack6/1
  Multiport Switch1/1 -> [LV_TC_Torque_Cmd]
  [LV_TC_Torque_Cmd] -> Rate Transition5/1
  [Knob2] -> Pedals Curve Switcher/1(Knob 2)
  [Screen] -> Pedals Curve Switcher/2(Screen)
  Rate Transition5/1 -> CAN Pack2/4
  From19/1 -> "Ki: 0-100 "/1
  [Knob1] -> Power Limiting/1(In1)
  Subsystem/1(Out1) -> Power Limiting/2(In2)
  Power Limiting/1(Out1) -> Min2/2
  Kalman Filter/4(Slip Ratio) -> [Slip_Ratio], Subsystem2/4(In4)
  [Rear_Speed] -> TC Controller 2/5(v_avg)
  [Fwd_Speed_Est] -> TC Controller 2/3(Forward Speed Estimate)
  [Slip_Ratio] -> TC Controller 2/4(Slip Ratio)
  [Slip_Ratio] -> TC Controller 1/1(k)
  [Fwd_Speed_Est] -> Rate Transition1/1
  [Lateral_Accel] -> Rate Transition2/1
  [Fwd_Accel] -> TC Controller 2/1(a_x)
  [Knob2] -> Min Torque %: 0.5-0.725/1
  Min Torque %: 0.5-0.725/1 -> TC Controller 2/9(Minimum Model Torque)
  Mu: 0.8-1.7/1 -> TC Controller 2/6(Driver u)
  Constant4/1 -> TC Controller 2/7(Kp)
  Constant5/1 -> TC Controller 2/8(Ki)
  [Driver_Torque] -> CAN Pack2/3
  GreaterThanOrEqual1/1 -> [Brake_Light]
  [Brake_Light] -> RT4/1
  [Brake_Light] -> CAN Pack5/1
  [Brake_Light] -> brake_light_mcu_60/1
  NOT1/1 -> AND2/1
  AND2/1 -> Green_Light/1
  Digital Clock2/1 -> MATLAB Function1/2(time)
  OR1/1 -> AND/2
  Hit Crossing/1 -> OR2/1
  Hit Crossing1/1 -> OR2/2
  OR2/1 -> MATLAB Function1/1(u)
  MATLAB Function1/1(y) -> NOT1/1, OR1/2
  NOT/1 -> OR1/1
  Pulse Generator/1 -> AND/1
  AND/1 -> Red_Light/1
  MATLAB Function9/2(r_faults) -> RT/1, Demux/1
  [Lateral_Accel] -> TC Controller 2/2(Lateral Accel)

== system main/Function-Call Subsystem ==
  In1 : Inport
  function : TriggerPort  TriggerType=function-call  VariantControl=(inherit)
  CAN Unpack : canmsglib/CAN Unpack  Commented=on  CANdbFile=C:\Users\Columbia\Documents\GitHub\EV24-Software\CAN\EV24 CAN.dbc  MsgList=(none)  MsgName=M002_TS_State  MsgIDType=Standard (11-bit identifier)  MsgIdentifier=2  MsgLength=1  SignalInfo={'ACC_TS_State','0','8','LE','signed','Standard','0','1','0','-Inf','Inf'}  IDPort=off  TimestampPort=off  ErrorPort=off  RemotePort=off  LengthPort=off  StatusPort=off  ApplyMinMax=off
      settings: DataFormat=CANdb specified signals
  CAN Unpack1 : canmsglib/CAN Unpack  MsgList=(none)  MsgName=M002_TS_State  MsgIDType=Standard (11-bit identifier)  MsgIdentifier=2  MsgLength=6  SignalInfo={ 'ACC_TS_State', '0', '8', 'LE', 'signed', 'Standard', '0', '1', '0', '-Inf', 'Inf' }  IDPort=off  TimestampPort=off  ErrorPort=off  RemotePort=off  LengthPort=off  StatusPort=off  ApplyMinMax=off
  Out1 : Outport  OutDataTypeStr=int8
  wires:
  CAN Unpack1/1 -> Out1/1
  In1/1 -> CAN Unpack1/1

== system main/Function-Call Subsystem1 ==
  In1 : Inport
  function : TriggerPort  TriggerType=function-call  VariantControl=(inherit)
  CAN Unpack : canmsglib/CAN Unpack  CANdbFile=C:\Users\lukeh\Documents\FSAE\EV24-Software\CAN\20240129 Gen5 CAN DB.dbc  MsgList=(none)  MsgName=M154_Internal_States  MsgIDType=Standard (11-bit identifier)  MsgIdentifier=154  MsgLength=8  SignalInfo={'INV_BMS_Active','57','1','LE','unsigned','Standard','0','1','0','0','1';'INV_BMS_Torque_Limiting','58','1','LE','unsigned','Standard','0','1','0','0','1';'INV_Burst_Model_Mode','49','1','LE','unsigned','Standard','0','1','0','0','1';'INV_Direction_Command','56','1','LE','unsigned','Standard','0','1','0','0','1';'INV_Inverter_Command_Mode','40','1','LE','unsigned','Standard','0','1','0','0','1';'INV_Inverter_Discharge_State','37','3','LE','unsigned','Standard','0','1','0','0','7';'INV_Inverter_Enable_Lockout','55','1','LE','unsigned','Standard','0','1','0','0','1';'INV_Inverter_Enable_State','48','1','LE','unsigned','Standard','0','1','0','0','1';'INV_Inverter_Run_Mode','32','1','LE','unsigned','Standard','0','1','0','0','1';'INV_Inverter_State','16','8','LE','unsigned','Standard','0','1','0','0','255';'INV_Key_Switch_Start_Status','54','1','LE','unsigned','Standard','0','1','0','0','1';'INV_Limit_Coolant_Derating','62','1','LE','unsigned','Standard','0','1','0','0','1';'INV_Limit_Hot_Spot','60','1','LE','unsigned','Standard','0','1','0','0','1';'INV_Limit_Max_Speed','59','1','LE','unsigned','Standard','0','1','0','0','1';'INV_Limit_Stall_Burst_Model','63','1','LE','unsigned','Standard','0','1','0','0','1';'INV_Low_Speed_Limiting','61','1','LE','unsigned','Standard','0','1','0','0','1';'INV_PWM_Frequency','8','8','LE','unsigned','Standard','0','1','0','0','255';'INV_Relay_1_Status','24','1','LE','unsigned','Standard','0','1','0','0','1';'INV_Relay_2_Status','25','1','LE','unsigned','Standard','0','1','0','0','1';'INV_Relay_3_Status','26','1','LE','unsigned','Standard','0','1','0','0','1';'INV_Relay_4_Status','27','1','LE','unsigned','Standard','0','1','0','0','1';'INV_Relay_5_Status','28','1','LE','unsigned','Standard','0','1','0','0','1';'INV_Relay_6_Status','29','1','LE','unsigned','Standard','0','1','0','0','1';'INV_Rolling_Counter','44','4','LE','unsigned','Standard','0','1','0','0','15';'INV_Self_Sensing_Assist_Enable','33','1','LE','unsigned','Standard','0','1','0','0','1';'INV_VSM_State','0','8','LE','unsigned','Standard','0','1','0','0','15'}  IDPort=off  TimestampPort=off  ErrorPort=off  RemotePort=off  LengthPort=off  StatusPort=off  ApplyMinMax=off
      settings: DataFormat=CANdb specified signals
  inv_en : Outport  OutDataTypeStr=uint8
  wires:
  In1/1 -> CAN Unpack/1
  CAN Unpack/8 -> inv_en/1

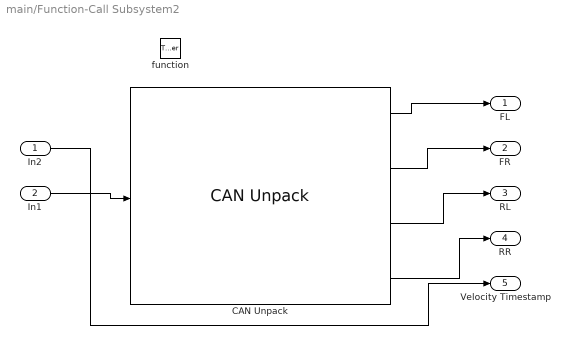
== system main/Function-Call Subsystem2 ==
  In2 : Inport
  In1 : Inport  Port=2
  function : TriggerPort  TriggerType=function-call  VariantControl=(inherit)
  CAN Unpack : canmsglib/CAN Unpack  MsgList=(none)  MsgName=M051_Wheel_Speeds  MsgIDType=Standard (11-bit identifier)  MsgIdentifier=51  MsgLength=8  SignalInfo={'SEN_WSS_FL','0','16','LE','unsigned','Standard','0','0.1','0','0','6553.5';'SEN_WSS_FR','16','16','LE','unsigned','Standard','0','0.1','0','0','163.8375';'SEN_WSS_RL','32','16','LE','unsigned','Standard','0','0.1','0','0','6553.5';'SEN_WSS_RR','48','16','LE','unsigned','Standard','0','0.1','0','0','6553.5'}  IDPort=off  TimestampPort=off  ErrorPort=off  RemotePort=off  LengthPort=off  StatusPort=off  ApplyMinMax=off
  FL : Outport  OutDataTypeStr=double
  FR : Outport  Port=2  OutDataTypeStr=double
  RL : Outport  Port=3  OutDataTypeStr=double
  RR : Outport  Port=4  OutDataTypeStr=double
  Velocity Timestamp : Outport  Port=5
  wires:
  In1/1 -> CAN Unpack/1
  CAN Unpack/1 -> FL/1
  CAN Unpack/4 -> RR/1
  CAN Unpack/2 -> FR/1
  CAN Unpack/3 -> RL/1
  In2/1 -> Velocity Timestamp/1

== system main/Function-Call Subsystem3 ==
  In1 : Inport
  In2 : Inport  Port=2
  function : TriggerPort  TriggerType=function-call  VariantControl=(inherit)
  CAN Unpack : canmsglib/CAN Unpack  MsgList=(none)  MsgName=M052_G_Forces  MsgIDType=Standard (11-bit identifier)  MsgIdentifier=52  MsgLength=6  SignalInfo={'SEN_G_FORCE_X','0','16','LE','signed','Standard','0','0.01','0','-327.68','327.67';'SEN_G_FORCE_Y','16','16','LE','signed','Standard','0','0.01','0','-327.68','327.67';'SEN_G_FORCE_Z','32','16','LE','signed','Standard','0','0.01','0','-327.68','327.67'}  IDPort=off  TimestampPort=off  ErrorPort=off  RemotePort=off  LengthPort=off  StatusPort=off  ApplyMinMax=off
  Accel from CAN : Outport  OutDataTypeStr=double
  Accel Report : Outport  Port=2
  Lateral Accel : Outport  Port=3
  wires:
  In1/1 -> CAN Unpack/1
  CAN Unpack/1 -> Accel from CAN/1
  CAN Unpack/2 -> Lateral Accel/1
  In2/1 -> Accel Report/1

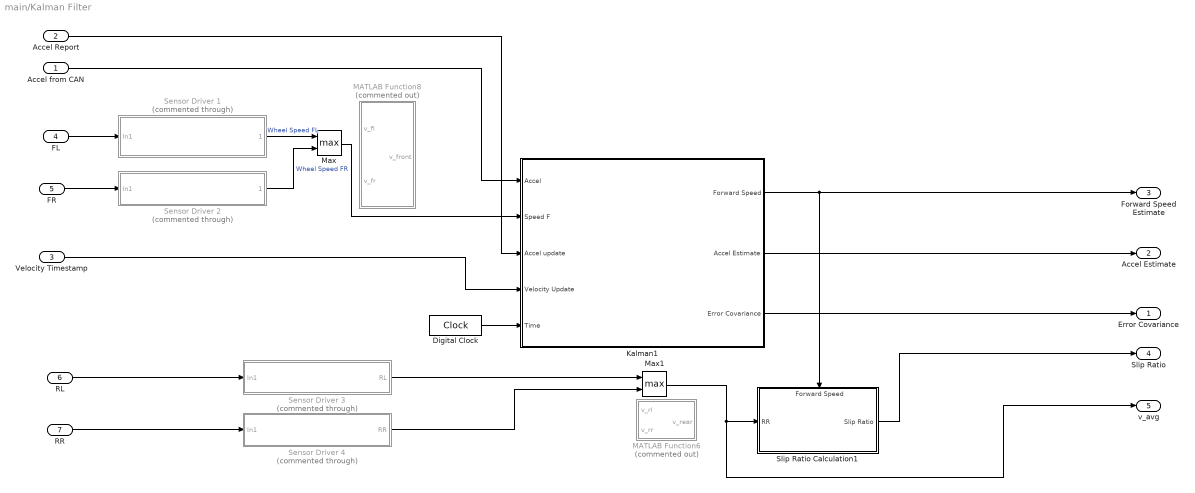
== system main/Kalman Filter ==
  Accel from CAN : Inport
  Accel Report : Inport  Port=2
  Velocity Timestamp : Inport  Port=3
  FL : Inport  Port=4
  FR : Inport  Port=5
  RL : Inport  Port=6
  RR : Inport  Port=7
  Digital Clock : DigitalClock  SampleTime=0.001
  Kalman1 : Subsystem
  MATLAB Function6 : MATLAB Function  Commented=on  TreatAsAtomicUnit=on
  MATLAB Function8 : MATLAB Function  Commented=on  TreatAsAtomicUnit=on
  Max : MinMax  Function=max  Inputs=2
  Max1 : MinMax  Function=max  Inputs=2
  Sensor Driver 1 : Subsystem  Commented=through
  Sensor Driver 2 : Subsystem  Commented=through
  Sensor Driver 3 : Subsystem  Commented=through
  Sensor Driver 4 : Subsystem  Commented=through
  Slip Ratio Calculation1 : Subsystem
      settings: PortSchema="{\"entries\":[{\"content\":{\"sides\":[{\"content\":{\"connectorIds\":[\"In1\"]},\"type\":\"ConnectorPlacement.EquallySpacedRectSide\",\"uuid\":\"061c82cd-7e9c-4a72-b965-43235230dad9\"},{\"content\":{\"connectorIds\":[\"Out1\"],\"side\":\"RIGHT\"},\"type\":\"ConnectorPlacement.EquallySpacedRectSide\",\"uuid\":\"899eaa50-1c30-4f77-9d66-a8daefd9f1e3\"},{\"content\":{\"connectorIds\":[\"In2\"],\"side\":\"TOP\"},\"type\":\"ConnectorPlacement.EquallySpacedRectSide\",\"uuid\":\"89c07a25-5c36-4b16-a58e-7fbb1fd4b8e3\"}]},\"type\":\"ConnectorPlacement.EquallySpacedConnector\",\"uuid\":\"4f00da10-bd17-48bb-8760-fc873e4c20ca\"}],\"packageUris\":[\"http://schema.mathworks.com/mf0/Connector/R2020b\"],\"version\":\"1.0\"}"
  Error Covariance : Outport
  Accel Estimate : Outport  Port=2
  Forward Speed Estimate : Outport  Port=3
  Slip Ratio : Outport  Port=4
  v_avg : Outport  Port=5
  wires:
  Kalman1/1(Forward Speed) -> Slip Ratio Calculation1/2(Forward Speed), Forward Speed Estimate/1
  Slip Ratio Calculation1/1(Slip Ratio) -> Slip Ratio/1
  FR/1 -> Sensor Driver 2/1(In1)
  Sensor Driver 4/1(RR) -> Max1/2
  Sensor Driver 2/1(" ") -> Max/2  "Wheel Speed FR"
  RL/1 -> Sensor Driver 3/1(In1)
  Sensor Driver 1/1(" ") -> Max/1  "Wheel Speed FL"
  FL/1 -> Sensor Driver 1/1(In1)
  Sensor Driver 3/1(RL) -> Max1/1
  Accel from CAN/1 -> Kalman1/1(Accel)
  RR/1 -> Sensor Driver 4/1(In1)
  Digital Clock/1 -> Kalman1/5(Time)
  Kalman1/2(Accel Estimate) -> Accel Estimate/1
  Kalman1/3(Error Covariance) -> Error Covariance/1
  Velocity Timestamp/1 -> Kalman1/4(Velocity Update)
  Accel Report/1 -> Kalman1/3(Accel update)
  Max/1 -> Kalman1/2(Speed F)
  Max1/1 -> Slip Ratio Calculation1/1(RR), v_avg/1

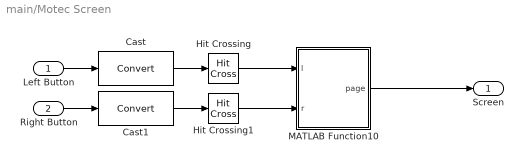
== system main/Motec Screen ==
  Left Button : Inport
  Right Button : Inport  Port=2
  Cast : DataTypeConversion  SaturateOnIntegerOverflow=off  RndMeth=Floor
  Cast1 : DataTypeConversion  SaturateOnIntegerOverflow=off  RndMeth=Floor
  Hit Crossing : HitCross  HitCrossingOffset=950  HitCrossingDirection=rising
  Hit Crossing1 : HitCross  HitCrossingOffset=950  HitCrossingDirection=rising
  MATLAB Function10 : MATLAB Function  TreatAsAtomicUnit=on
  Screen : Outport
  wires:
  Right Button/1 -> Cast1/1
  Left Button/1 -> Cast/1
  MATLAB Function10/1(page) -> Screen/1
  Hit Crossing/1 -> MATLAB Function10/1(l)
  Hit Crossing1/1 -> MATLAB Function10/2(r)
  Cast/1 -> Hit Crossing/1
  Cast1/1 -> Hit Crossing1/1

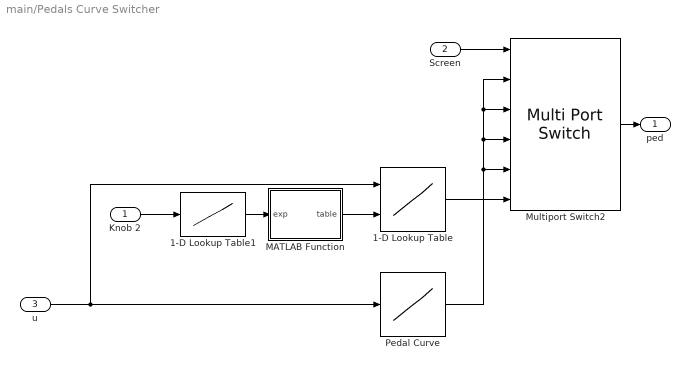
== system main/Pedals Curve Switcher ==
  Knob 2 : Inport
  Screen : Inport  Port=2
  u : Inport  Port=3
  1-D Lookup Table : Lookup_n-D  NumberOfTableDimensions=1  BreakpointsForDimension1=linspace(0,1,100)  TableSource=Input port  Table=linspace(0,1,100).^1.5  InternalRulePriority=Speed  RndMeth=Simplest
      settings: InputPortMap=u0,p221
  1-D Lookup Table1 : Lookup_n-D  NumberOfTableDimensions=1  BreakpointsForDimension1=[1 10]  Table=[1 5.5]  InternalRulePriority=Speed  RndMeth=Simplest
  MATLAB Function : MATLAB Function  TreatAsAtomicUnit=on
  Multiport Switch2 : MultiPortSwitch  DataPortOrder=Zero-based contiguous  Inputs=4  DataPortForDefault=Additional data port  zeroidx=on  SaturateOnIntegerOverflow=off  InputSameDT=off
  Pedal Curve : Lookup_n-D  NumberOfTableDimensions=1  BreakpointsForDimension1=[0 1]  Table=[0 1]  ExtrapMethod=Clip  UseLastTableValue=on  InternalRulePriority=Speed  RndMeth=Simplest
  ped : Outport
  wires:
  u/1 -> Pedal Curve/1, 1-D Lookup Table/1
  Pedal Curve/1 -> Multiport Switch2/2, Multiport Switch2/3, Multiport Switch2/4, Multiport Switch2/5
  1-D Lookup Table/1 -> Multiport Switch2/6
  Multiport Switch2/1 -> ped/1
  Knob 2/1 -> 1-D Lookup Table1/1
  MATLAB Function/1(table) -> 1-D Lookup Table/2
  1-D Lookup Table1/1 -> MATLAB Function/1(exp)
  Screen/1 -> Multiport Switch2/1

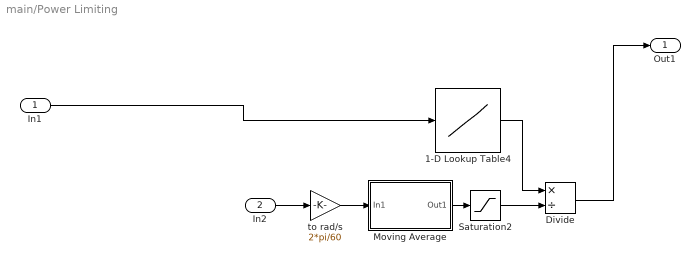
== system main/Power Limiting ==
  In1 : Inport
  In2 : Inport  Port=2
  1-D Lookup Table4 : Lookup_n-D  NumberOfTableDimensions=1  BreakpointsForDimension1=[1;10]  Table=[10e3;80e3]  ExtrapMethod=Clip  InternalRulePriority=Speed  RndMeth=Simplest
  Divide : Product  Inputs=*/
  Moving Average : Subsystem
  Saturation2 : Saturate  UpperLimit=inf  LowerLimit=1
  to rad/s : Gain  Gain=2*pi/60
  Out1 : Outport
  wires:
  Divide/1 -> Out1/1
  to rad/s/1 -> Moving Average/1(In1)
  Moving Average/1(Out1) -> Saturation2/1
  Saturation2/1 -> Divide/2
  1-D Lookup Table4/1 -> Divide/1
  In1/1 -> 1-D Lookup Table4/1
  In2/1 -> to rad/s/1

== system main/Subsystem ==
  In1 : Inport
  function : TriggerPort  TriggerType=function-call  VariantControl=(inherit)
  CAN Unpack : canmsglib/CAN Unpack  MsgList=(none)  MsgName=M149_Motor_Position_Info  MsgIDType=Standard (11-bit identifier)  MsgIdentifier=149  MsgLength=8  SignalInfo={'INV_Delta_Resolver_Filtered','48','16','LE','signed','Standard','0','0.1','0','-3276.8','3276.7';'INV_Electrical_Output_Frequency','32','16','LE','signed','Standard','0','0.1','0','-3276.8','3276.7';'INV_Motor_Angle_Electrical','0','16','LE','unsigned','Standard','0','0.1','0','0','6553.5';'INV_Motor_Speed','16','16','LE','signed','Standard','0','1','0','-32768','32767'}  IDPort=off  TimestampPort=off  ErrorPort=off  RemotePort=off  LengthPort=off  StatusPort=off  ApplyMinMax=off
      settings: LibrarySourceBlock=c2000lib/Target Communication/CAN Unpack
  Out1 : Outport
  wires:
  CAN Unpack/4 -> Out1/1
  In1/1 -> CAN Unpack/1

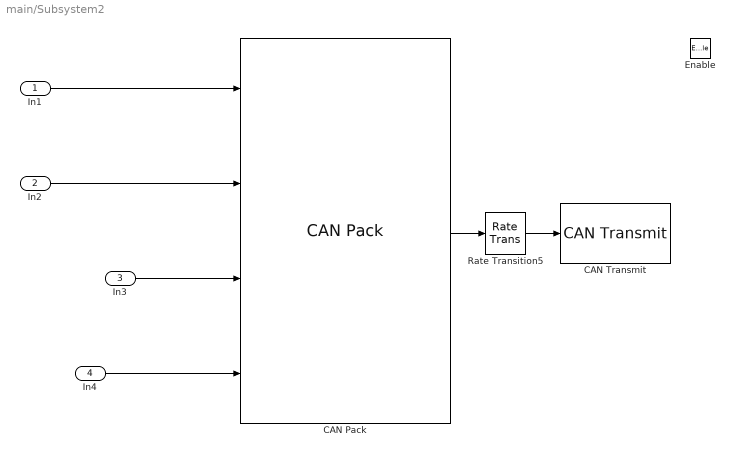
== system main/Subsystem2 ==
  In1 : Inport
  In2 : Inport  Port=2
  In3 : Inport  Port=3
  In4 : Inport  Port=4
  Enable : EnablePort
  CAN Pack : canmsglib/CAN Pack  MsgList=(none)  MsgName=M404_LV_Kalman_Outputs  MsgIDType=Standard (11-bit identifier)  MsgIdentifier=404  MsgLength=8  Remote=off  ApplyMinMax=off  BusOutput=off  SignalInfo={'LV_COV_V','32','16','LE','unsigned','Standard','0','0.02','0','0','1310.7';'LV_FILTERED_A','16','16','LE','signed','Standard','0','0.01','0','-327.68','327.67';'LV_FILTERED_V','0','16','LE','unsigned','Standard','0','0.1','0','0','6553.5';'LV_SR','48','16','LE','signed','Standard','0','0.0001','0','-3.2768','3.2767'}
      settings: LibrarySourceBlock=c2000lib/Target Communication/CAN Pack  DataFormat=manually specified signals
  CAN Transmit : c280xlib/CAN Transmit  chipFamily=C280x  useModule=CAN_B  mailboxNo=11  messageID=404  messageType=Standard (11-bit identifier)  enableBlockingMode=off  postInterrupt=off  interruptLine=0
  Rate Transition5 : RateTransition  OutPortSampleTime=0.05
  wires:
  CAN Pack/1 -> Rate Transition5/1
  In3/1 -> CAN Pack/3
  Rate Transition5/1 -> CAN Transmit/1
  In4/1 -> CAN Pack/4
  In2/1 -> CAN Pack/2
  In1/1 -> CAN Pack/1
